simulink library "microwave_class_defs"  (R2015a)
settings: Solver=ode45  StartTime=0.0  StopTime=10.0  RelTol=1e-3
libraries: sldvlib x2, microwave_class_defs x2, simulink x1
settings Model: Creator=Whalen  LastModifiedBy=Whalen
settings DebuggingCC: UnderspecifiedInitializationDetection=Classic  MergeDetectMultiDrivingBlocksExec=none  SolverPrmCheckMsg=warning  StateNameClashWarn=warning

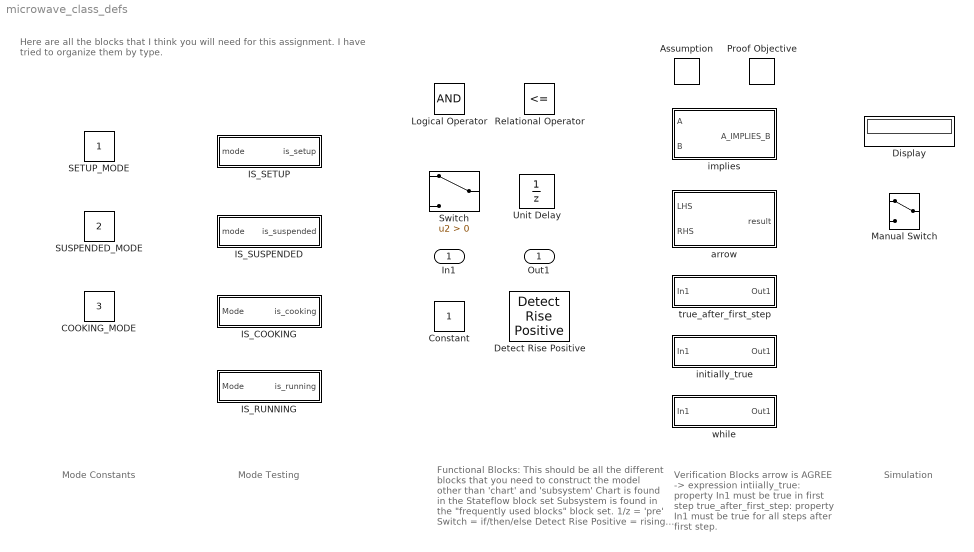
== system microwave_class_defs ==
  note: Here are all the blocks that I think you will need for this assignment.
      | I have tried to organize them by type.
  note: Mode Constants
  note: Mode Testing
  note: Verification Blocks
      |
      | arrow is AGREE -> expression
      | intiially_true: property In1 must
      |   be true in first step
      | true_after_first_step: property
      |   In1 must be true for all steps
      |   after first step.
  note: Functional Blocks: This
      | should be all the different blocks
      | that you need to construct the model
      | other than 'chart' and 'subsystem'
      |
      | Chart is found in the Stateflow block set
      | Subsystem is found in the "frequently used
      | blocks" block set.
      |
      | 1/z = 'pre'
      | Switch = if/then/else
      | Detect Rise Positive = rising edge
  note: Simulation
  In1 : Inport
  Assumption : sldvlib/Objectives and Constraints/Assumption  enabled=on  customAVTBlockType=Assumption  intervals=true  initial=off  dispValues=on  outEnabled=on
      settings: AttributesFormatString=%<intervals>
  COOKING_MODE : Constant  Value=3  OutDataTypeStr=uint8
  Constant : Constant
  Detect Rise Positive : simulink/Logic and Bit Operations/Detect Rise Positive  vinit=0  InputProcessing=Inherited  OutDataTypeStr=boolean
  Display : Display
  IS_COOKING : Subsystem
  IS_RUNNING : Subsystem
  IS_SETUP : Subsystem
  IS_SUSPENDED : Subsystem
  Logical Operator : Logic  AllPortsSameDT=off  OutDataTypeStr=boolean
  Manual Switch : ManualSwitch
  Proof Objective : sldvlib/Objectives and Constraints/Proof Objective  enabled=on  customAVTBlockType=Proof Objective  intervals=true  dispValues=on  outEnabled=on  enableStopSim=off
      settings: AttributesFormatString=%<intervals>
  Relational Operator : RelationalOperator  Operator=<=  OutDataTypeStr=boolean
  SETUP_MODE : Constant  OutDataTypeStr=uint8
  SUSPENDED_MODE : Constant  Value=2  OutDataTypeStr=uint8
  Switch : Switch  Criteria=u2 > Threshold
  Unit Delay : UnitDelay  SampleTime=-1
  arrow : Subsystem
  implies : Subsystem
  initially_true : Subsystem
  true_after_first_step : Subsystem
  while : Subsystem
  Out1 : Outport

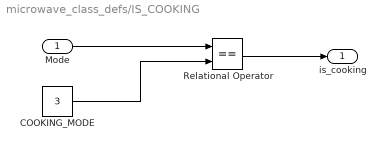
== system microwave_class_defs/IS_COOKING ==
  Mode : Inport  OutDataTypeStr=uint8
  COOKING_MODE : Constant  Value=3  OutDataTypeStr=uint8
  Relational Operator : RelationalOperator  Operator===  OutDataTypeStr=boolean
  is_cooking : Outport  OutDataTypeStr=boolean
  wires:
  Relational Operator/1 -> is_cooking/1
  COOKING_MODE/1 -> Relational Operator/2
  Mode/1 -> Relational Operator/1

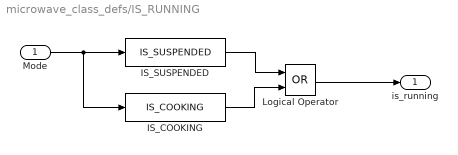
== system microwave_class_defs/IS_RUNNING ==
  Mode : Inport  OutDataTypeStr=uint8
  IS_COOKING : microwave_class_defs/IS_COOKING
  IS_SUSPENDED : microwave_class_defs/IS_SUSPENDED
  Logical Operator : Logic  Operator=OR  AllPortsSameDT=off  OutDataTypeStr=boolean
  is_running : Outport  OutDataTypeStr=boolean
  wires:
  Mode/1 -> IS_COOKING/1, IS_SUSPENDED/1
  Logical Operator/1 -> is_running/1
  IS_SUSPENDED/1 -> Logical Operator/1
  IS_COOKING/1 -> Logical Operator/2

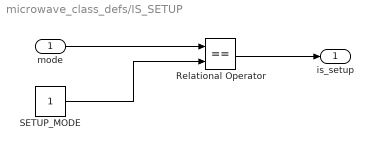
== system microwave_class_defs/IS_SETUP ==
  mode : Inport  OutDataTypeStr=uint8
  Relational Operator : RelationalOperator  Operator===  OutDataTypeStr=boolean
  SETUP_MODE : Constant  OutDataTypeStr=uint8
  is_setup : Outport  OutDataTypeStr=boolean
  wires:
  Relational Operator/1 -> is_setup/1
  SETUP_MODE/1 -> Relational Operator/2
  mode/1 -> Relational Operator/1

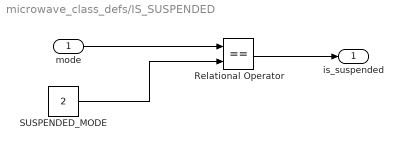
== system microwave_class_defs/IS_SUSPENDED ==
  mode : Inport  OutDataTypeStr=uint8
  Relational Operator : RelationalOperator  Operator===  OutDataTypeStr=boolean
  SUSPENDED_MODE : Constant  Value=2  OutDataTypeStr=uint8
  is_suspended : Outport  OutDataTypeStr=boolean
  wires:
  mode/1 -> Relational Operator/1
  SUSPENDED_MODE/1 -> Relational Operator/2
  Relational Operator/1 -> is_suspended/1

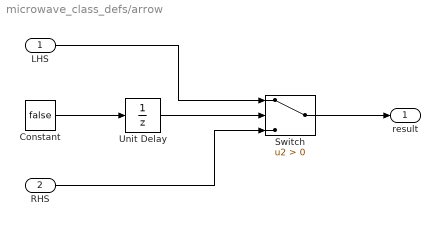
== system microwave_class_defs/arrow ==
  LHS : Inport
  RHS : Inport  Port=2
  Constant : Constant  Value=false  OutDataTypeStr=boolean
  Switch : Switch  Criteria=u2 > Threshold
  Unit Delay : UnitDelay  InitialCondition=true  SampleTime=-1
  result : Outport
  wires:
  Constant/1 -> Unit Delay/1
  LHS/1 -> Switch/1
  Unit Delay/1 -> Switch/2
  RHS/1 -> Switch/3
  Switch/1 -> result/1

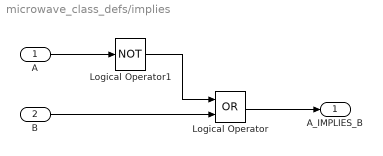
== system microwave_class_defs/implies ==
  A : Inport
  B : Inport  Port=2
  Logical Operator : Logic  Operator=OR  AllPortsSameDT=off  OutDataTypeStr=boolean
  Logical Operator1 : Logic  Operator=NOT  AllPortsSameDT=off  OutDataTypeStr=boolean
  A_IMPLIES_B : Outport
  wires:
  A/1 -> Logical Operator1/1
  B/1 -> Logical Operator/2
  Logical Operator1/1 -> Logical Operator/1
  Logical Operator/1 -> A_IMPLIES_B/1

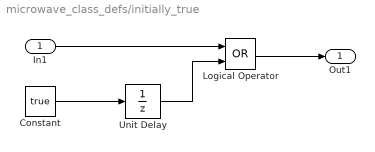
== system microwave_class_defs/initially_true ==
  In1 : Inport
  Constant : Constant  Value=true  OutDataTypeStr=boolean
  Logical Operator : Logic  Operator=OR  AllPortsSameDT=off  OutDataTypeStr=boolean
  Unit Delay : UnitDelay  InitialCondition=false  SampleTime=-1
  Out1 : Outport
  wires:
  Logical Operator/1 -> Out1/1
  In1/1 -> Logical Operator/1
  Unit Delay/1 -> Logical Operator/2
  Constant/1 -> Unit Delay/1

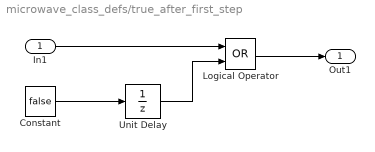
== system microwave_class_defs/true_after_first_step ==
  In1 : Inport
  Constant : Constant  Value=false  OutDataTypeStr=boolean
  Logical Operator : Logic  Operator=OR  AllPortsSameDT=off  OutDataTypeStr=boolean
  Unit Delay : UnitDelay  InitialCondition=true  SampleTime=-1
  Out1 : Outport
  wires:
  Constant/1 -> Unit Delay/1
  Unit Delay/1 -> Logical Operator/2
  In1/1 -> Logical Operator/1
  Logical Operator/1 -> Out1/1

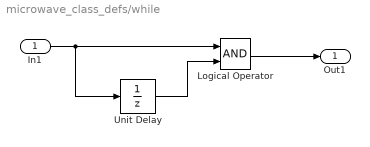
== system microwave_class_defs/while ==
  In1 : Inport
  Logical Operator : Logic  AllPortsSameDT=off  OutDataTypeStr=boolean
  Unit Delay : UnitDelay  InitialCondition=false  SampleTime=-1
  Out1 : Outport
  wires:
  In1/1 -> Unit Delay/1, Logical Operator/1
  Unit Delay/1 -> Logical Operator/2
  Logical Operator/1 -> Out1/1
